simulink model "redgreenyellowyahoomario"  (R2023a)
settings: Solver=FixedStepAuto  StartTime=0.0  StopTime=30  FixedStep=1  RelTol=1e-3
libraries: simulink x6
settings Model: Creator=s3979639  LastModifiedBy=s3979639

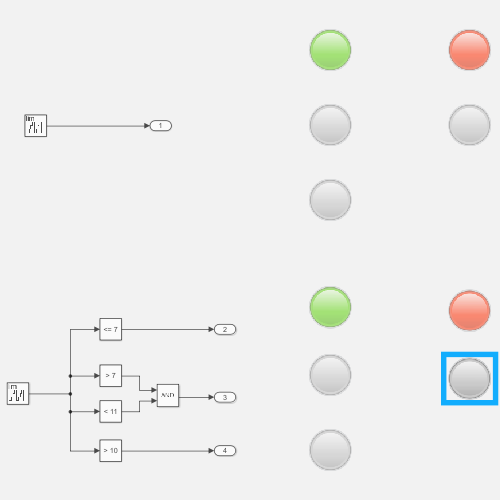
[thumbnail: Simulink's stored preview of the top-level diagram]
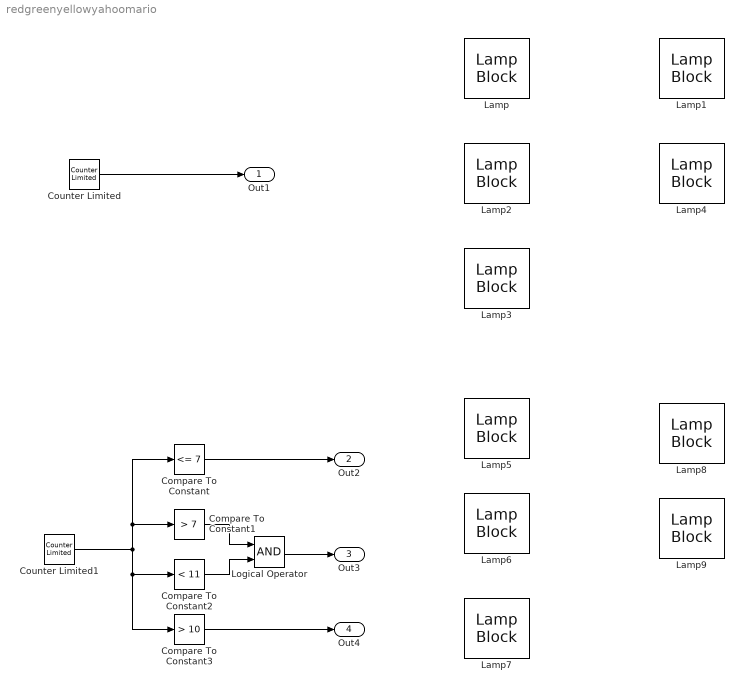
== system redgreenyellowyahoomario ==
  Compare To Constant : simulink/Logic and Bit Operations/Compare To Constant  relop=<=  const=7  OutDataTypeStr=boolean
  Compare To Constant1 : simulink/Logic and Bit Operations/Compare To Constant  relop=>  const=7  OutDataTypeStr=boolean
  Compare To Constant2 : simulink/Logic and Bit Operations/Compare To Constant  relop=<  const=11  OutDataTypeStr=boolean
  Compare To Constant3 : simulink/Logic and Bit Operations/Compare To Constant  relop=>  const=10  OutDataTypeStr=boolean
  Counter Limited : simulink/Sources/Counter Limited  uplimit=15  tsamp=-1
  Counter Limited1 : simulink/Sources/Counter Limited  uplimit=15  tsamp=-1
  Lamp{,1..9} (10 alike) : LampBlock  LabelPosition=Hide
  Logical Operator : Logic  AllPortsSameDT=off  OutDataTypeStr=boolean
  Out1 : Outport
  Out2 : Outport  Port=2
  Out3 : Outport  Port=3
  Out4 : Outport  Port=4
  wires:
  Counter Limited/1 -> Out1/1
  Counter Limited1/1 -> Compare To Constant3/1, Compare To Constant2/1, Compare To Constant1/1, Compare To Constant/1
  Compare To Constant1/1 -> Logical Operator/1
  Compare To Constant2/1 -> Logical Operator/2
  Compare To Constant/1 -> Out2/1
  Logical Operator/1 -> Out3/1
  Compare To Constant3/1 -> Out4/1
